simulink model "Contoh_Phoebe_2_noswitch_FIX"  (R2020b)
settings: Solver=VariableStepAuto  StartTime=0.0  StopTime=110000  FixedStep=1  RelTol=1e-3  EnableMultiTasking=on
PostLoadFcn:
  | a=find_system(gcs,'Name','Figure 1');
  | set_param(a{1},'Open','on');
  | shh = get(0,'ShowHiddenHandles');
  | set(0,'ShowHiddenHandles','On');
  | set(gcf,'Position',[500   280   546   449]);
  | set(0,'ShowHiddenHandles',shh);
InitFcn:
  | load datazr;
  | load datazl;
values from neighbouring files (symbols this model uses):
  G = 0.4*1e-5    (= 4e-06)    [initrun.m]
  k1 = 2*ze*wn*I/G    [initrun.m]
  k2 = 1    [initrun.m]
undefined symbols (not defined in the file or in its folder): gcf, outputDelta, pCalc, semimajor, set, Zl, Zr
libraries: aerolibconvert2 x2, vrlib x2, simulink x1
settings Model: Creator=Ridanto  LastModifiedBy=Asus
settings SolverCC: ZeroCrossAlgorithm=Adaptive
settings DataIOCC: LimitDataPoints=on  SaveFormat=Array  SignalLoggingSaveFormat=ModelDataLogs  ReturnWorkspaceOutputs=off
settings OptimizationCC: BufferReuse=off  ExpressionDepthLimit=2147483647  InitFltsAndDblsToZero=on  LifeSpan=inf
settings DebuggingCC: SaveWithParameterizedLinksMsg=none  UnderspecifiedInitializationDetection=Classic  MergeDetectMultiDrivingBlocksExec=none  SignalResolutionControl=TryResolveAllWithWarning  IgnoredZcDiagnostic=none  SolverPrmCheckMsg=warning  MultiTaskDSMMsg=warning  MultiTaskCondExecSysMsg=none  FcnCallInpInsideContextMsg=warning  StateNameClashWarn=warning  SFUnexpectedBacktrackingDiag=warning  SFNoUnconditionalDefaultTransitionDiag=warning  SFExecutionAtInitializationDiag=none  ArithmeticOperatorsInVariantConditions=warning
settings HardwareCC: ProdBitPerPointer=32  ProdBitPerSizeT=32  ProdBitPerPtrDiffT=32  ProdLargestAtomicFloat=None  ProdIntDivRoundTo=Undefined  ProdEndianess=Unspecified  ProdWordSize=32  ProdHWDeviceType=32-bit Generic
settings ModelReferenceCC: PropagateSignalLabelsOutOfModel=off
settings SFSimCC: SimUseLocalCustomCode=off  SimParseCustomCode=off  CustomCodeUndefinedFunction=UseInterfaceOnly
settings RTWCC: RTWUseLocalCustomCode=off
settings CodeAppCC: StateflowObjectComments=on
settings GRTTargetCC: TargetFcnLib=ansi_tfl_tmw.mat  TargetLangStandard=C89/C90 (ANSI)  CombineOutputUpdateFcns=off  GRTInterface=on
settings ConfigComp: CovMetricSettings=dw  CovSaveCumulativeToWorkspaceVar=on  CovSaveSingleToWorkspaceVar=on  CovExternalEMLEnable=off
settings SimscapeCC: SimscapeNormalizeSystem=off
settings ConfigurationSet: Description=SimMechanics 2G

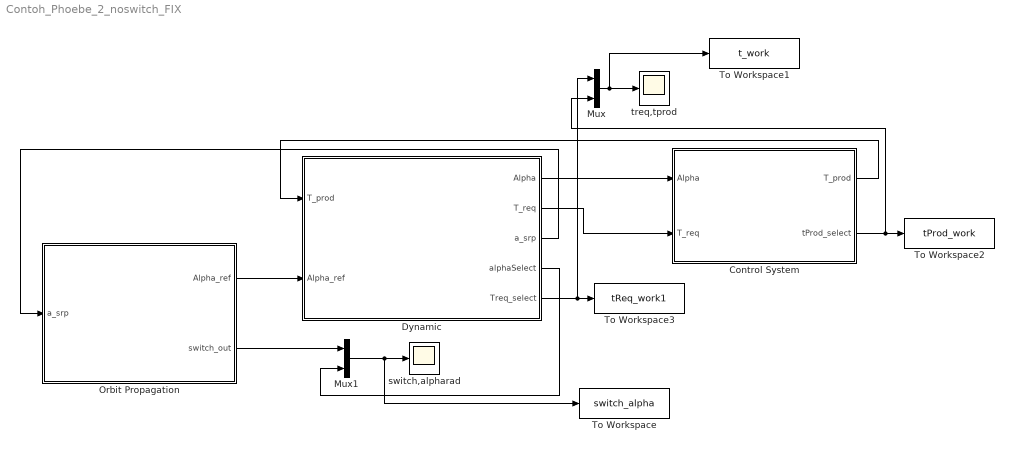
== system Contoh_Phoebe_2_noswitch_FIX ==
  Control System : Subsystem
  Dynamic : Subsystem
  Mux : Mux  Inputs=2
  Mux1 : Mux  Inputs=2
  Orbit Propagation : Subsystem
  To Workspace : ToWorkspace  VariableName=switch_alpha  SaveFormat=Timeseries  SampleTime=-1
  To Workspace1 : ToWorkspace  VariableName=t_work  SaveFormat=Timeseries  SampleTime=-1
  To Workspace2 : ToWorkspace  VariableName=tProd_work  SaveFormat=Timeseries  SampleTime=-1
  To Workspace3 : ToWorkspace  VariableName=tReq_work1  SaveFormat=Timeseries  SampleTime=-1
  switch,alpharad : Scope
  treq,tprod : Scope
  wires:
  Dynamic/2(T_req) -> Control System/2(T_req)
  Dynamic/3(a_srp) -> Orbit Propagation/1(a_srp)
  Dynamic/1(Alpha) -> Control System/1(Alpha)
  Orbit Propagation/1(Alpha_ref) -> Dynamic/2(Alpha_ref)
  Control System/1(T_prod) -> Dynamic/1(T_prod)
  Mux1/1 -> To Workspace/1, switch,alpharad/1
  Orbit Propagation/2(switch_out) -> Mux1/1
  Dynamic/4(alphaSelect) -> Mux1/2
  Mux/1 -> To Workspace1/1, treq,tprod/1
  Control System/2(tProd_select) -> Mux/2, To Workspace2/1
  Dynamic/5(Treq_select) -> Mux/1, To Workspace3/1

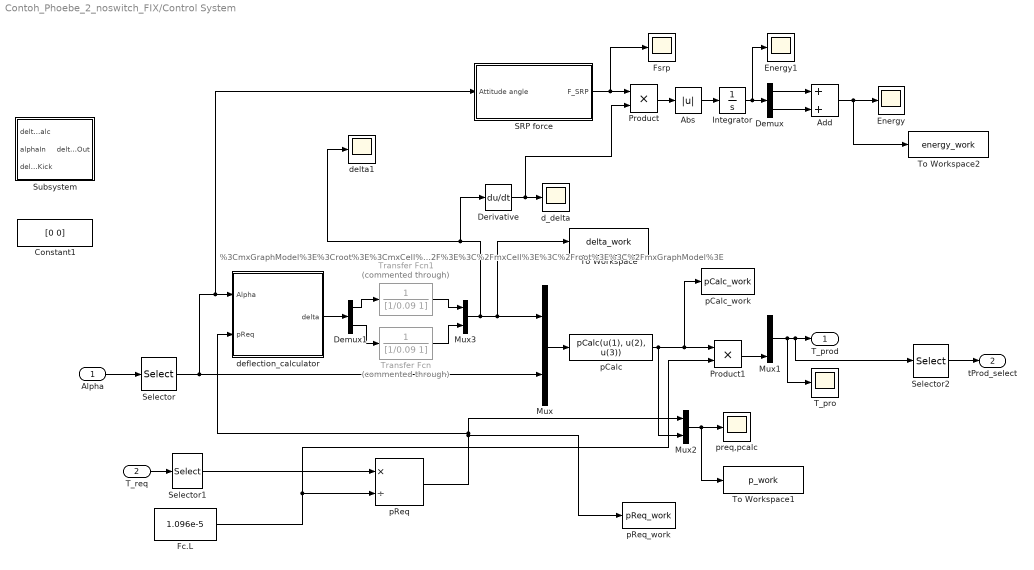
== system Contoh_Phoebe_2_noswitch_FIX/Control System ==
  note: %3CmxGraphModel%3E%3Croot%3E%3CmxCell%20id%3D%220%22%2F%3E%3CmxCell%20id%3D%221%22%20parent%3D%220%22%2F%3E%3CmxCell%20id%3D%222%22%20value%3D%22A%22%20style%3D%22ellipse%3BwhiteSpace%3Dwrap%3Bhtml%3D1%3Baspect%3Dfixed%3BfillColor%3Dnone%3B%22%20vertex%3D%221%22%20parent%3D%221%22%3E%3CmxGeometry%20x%3D%22170%22%20y%3D%221331%22%20width%3D%2260%22%20height%3D%2260%22%20as%3D%22geometry%22%2F%3E%3C%2FmxCell%3E%3C%2Froot%3E%3C%2FmxGraphModel%3E
  Alpha : Inport
  T_req : Inport  Port=2
  Abs : Abs
  Add : Sum
  Constant1 : Constant  Value=[0 0]
  Demux : Demux  Outputs=2
  Demux1 : Demux  Outputs=2
  Derivative : Derivative
  Energy : Scope
  Energy1 : Scope
  Fc.L : Constant  Value=1.096e-5
  Fsrp : Scope
  Integrator : Integrator
  Mux : Mux  Inputs=2
  Mux1 : Mux  Inputs=3
  Mux2 : Mux  Inputs=2
  Mux3 : Mux  Inputs=2
  Product : Product
  Product1 : Product
  SRP force : Subsystem
  Selector : Selector  InputPortWidth=3  IndexOptions=Index vector (dialog)  Indices=3  OutputSizes=1
  Selector1 : Selector  InputPortWidth=3  IndexOptions=Index vector (dialog)  Indices=3  OutputSizes=1
  Selector2 : Selector  InputPortWidth=3  IndexOptions=Index vector (dialog)  Indices=3  OutputSizes=1
  Subsystem : Subsystem
  T_pro : Scope
  To Workspace : ToWorkspace  VariableName=delta_work  SaveFormat=Timeseries  SampleTime=-1
  To Workspace1 : ToWorkspace  VariableName=p_work  SaveFormat=Timeseries  SampleTime=-1
  To Workspace2 : ToWorkspace  VariableName=energy_work  SaveFormat=Timeseries  SampleTime=-1
  Transfer Fcn : TransferFcn  Commented=through  Denominator=[1/0.09 1]
  Transfer Fcn1 : TransferFcn  Commented=through  Denominator=[1/0.09 1]
  d_delta : Scope
  deflection_calculator : Subsystem
  delta1 : Scope
  pCalc : MATLABFcn  MATLABFcn=pCalc(u(1), u(2), u(3))  OutputDimensions=1
  pCalc_work : ToWorkspace  VariableName=pCalc_work  SaveFormat=Timeseries  SampleTime=-1
  pReq : Product  Inputs=*/
  pReq_work : ToWorkspace  VariableName=pReq_work  SaveFormat=Timeseries  SampleTime=-1
  preq,pcalc : Scope
  T_prod : Outport
  tProd_select : Outport  Port=2
  wires:
  pReq/1 -> deflection_calculator/2(pReq), Mux2/1, pReq_work/1
  Mux1/1 -> Selector2/1, T_prod/1, T_pro/1
  Selector/1 -> Mux/2, deflection_calculator/1(Alpha), SRP force/1(Attitude angle)
  pCalc/1 -> Mux2/2, pCalc_work/1, Product1/1
  Product1/1 -> Mux1/3
  Fc.L/1 -> pReq/2, Product1/2
  Mux2/1 -> To Workspace1/1, preq,pcalc/1
  T_req/1 -> Selector1/1
  Alpha/1 -> Selector/1
  Mux/1 -> pCalc/1
  Selector1/1 -> pReq/1
  Derivative/1 -> Product/2, d_delta/1
  SRP force/1(F_SRP) -> Fsrp/1, Product/1
  Integrator/1 -> Energy1/1, Demux/1
  Demux/1 -> Add/1
  Demux/2 -> Add/2
  Add/1 -> To Workspace2/1, Energy/1
  Selector2/1 -> tProd_select/1
  Product/1 -> Abs/1
  Abs/1 -> Integrator/1
  deflection_calculator/1(delta) -> Demux1/1
  Demux1/2 -> Transfer Fcn/1
  Demux1/1 -> Transfer Fcn1/1
  Transfer Fcn1/1 -> Mux3/1
  Transfer Fcn/1 -> Mux3/2
  Mux3/1 -> delta1/1, Derivative/1, To Workspace/1, Mux/1

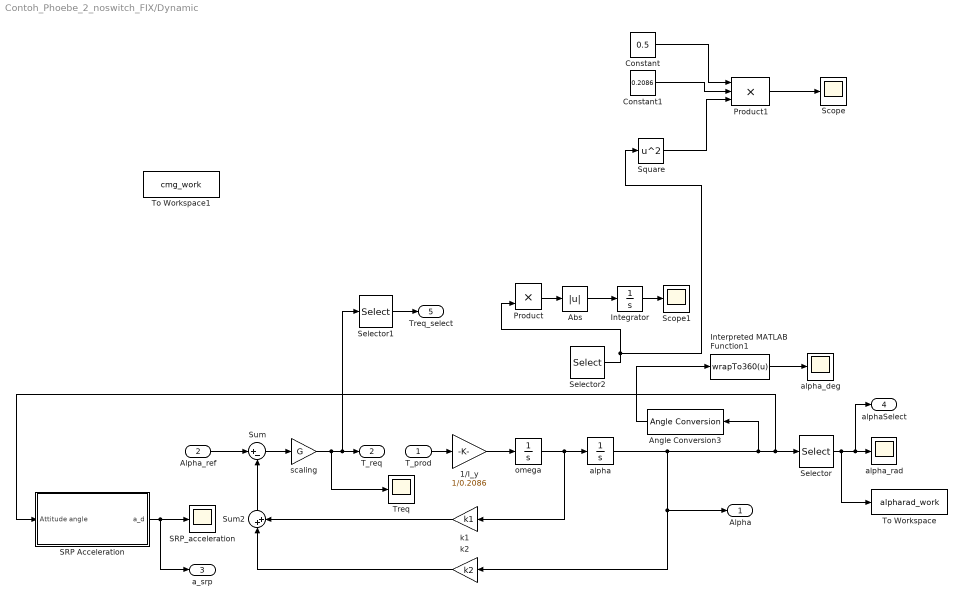
== system Contoh_Phoebe_2_noswitch_FIX/Dynamic ==
  T_prod : Inport
  Alpha_ref : Inport  Port=2
  1/I_y : Gain  Gain=1/0.2086
  Abs : Abs
  Angle Conversion3 : aerolibconvert2/Angle Conversion  IU=rad  OU=deg
  Constant : Constant  Value=0.5
  Constant1 : Constant  Value=0.2086
  Integrator : Integrator
  Interpreted MATLAB Function1 : MATLABFcn  MATLABFcn=wrapTo360(u)  OutputDimensions=3
  Product : Product
  Product1 : Product  Inputs=3
  SRP Acceleration : Subsystem
  SRP_acceleration : Scope
  Scope : Scope
  Scope1 : Scope
  Selector : Selector  InputPortWidth=3  IndexOptions=Index vector (dialog)  Indices=3  OutputSizes=1
  Selector1 : Selector  InputPortWidth=3  IndexOptions=Index vector (dialog)  Indices=3  OutputSizes=1
  Selector2 : Selector  InputPortWidth=3  IndexOptions=Index vector (dialog)  Indices=3  OutputSizes=1
  Square : Math  Operator=square  SaturateOnIntegerOverflow=on
  Sum : Sum  Inputs=|+-
  Sum2 : Sum  Inputs=|++
  To Workspace : ToWorkspace  VariableName=alpharad_work  SaveFormat=Timeseries  SampleTime=-1
  To Workspace1 : ToWorkspace  VariableName=cmg_work  SaveFormat=Timeseries  SampleTime=-1
  Treq : Scope
  alpha : Integrator  WrapState=on
  alpha_deg : Scope
  alpha_rad : Scope
  k1 : Gain  Gain=k1
  k2 : Gain  Gain=k2
  omega : Integrator
  scaling : Gain  Gain=G
  Alpha : Outport
  T_req : Outport  Port=2
  a_srp : Outport  Port=3
  alphaSelect : Outport  Port=4
  Treq_select : Outport  Port=5
  wires:
  Interpreted MATLAB Function1/1 -> alpha_deg/1
  k2/1 -> Sum2/1
  Sum2/1 -> Sum/2
  SRP Acceleration/1(a_d) -> a_srp/1, SRP_acceleration/1
  1/I_y/1 -> omega/1
  k1/1 -> Sum2/2
  Angle Conversion3/1 -> Interpreted MATLAB Function1/1
  Alpha_ref/1 -> Sum/1
  Sum/1 -> scaling/1
  alpha/1 -> Selector/1, SRP Acceleration/1(Attitude angle), Angle Conversion3/1, Alpha/1, k2/1
  Selector/1 -> To Workspace/1, alphaSelect/1, alpha_rad/1
  Selector1/1 -> Treq_select/1
  scaling/1 -> T_req/1, Selector1/1, Treq/1
  omega/1 -> alpha/1, k1/1
  Constant1/1 -> Product1/2
  Constant/1 -> Product1/1
  Product1/1 -> Scope/1
  Square/1 -> Product1/3
  Abs/1 -> Integrator/1
  Product/1 -> Abs/1
  Integrator/1 -> Scope1/1
  Selector2/1 -> Square/1, Product/2
  T_prod/1 -> 1/I_y/1

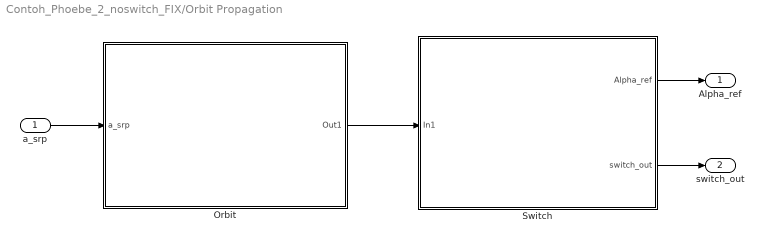
== system Contoh_Phoebe_2_noswitch_FIX/Orbit Propagation ==
  a_srp : Inport
  "Orbit " : Subsystem
  Switch : Subsystem
  Alpha_ref : Outport
  switch_out : Outport  Port=2
  wires:
  "Orbit "/1(Out1) -> Switch/1(In1)
  a_srp/1 -> "Orbit "/1(a_srp)
  Switch/1(Alpha_ref) -> Alpha_ref/1
  Switch/2(switch_out) -> switch_out/1

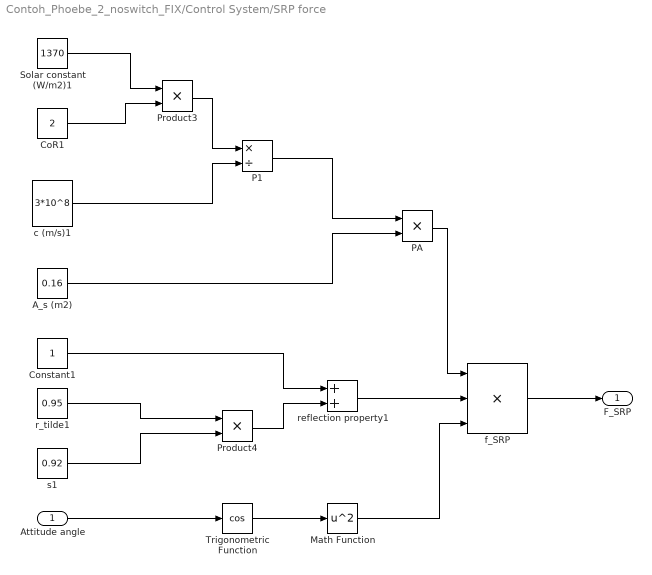
== system Contoh_Phoebe_2_noswitch_FIX/Control System/SRP force ==
  Attitude angle : Inport
  A_s (m2) : Constant  Value=0.16
  CoR1 : Constant  Value=2
  Constant1 : Constant
  Math Function : Math  Operator=square  SaturateOnIntegerOverflow=on
  P1 : Product  Inputs=*/
  PA : Product
  Product3 : Product
  Product4 : Product
  Solar constant (W/m2)1 : Constant  Value=1370
  Trigonometric Function : Trigonometry  Operator=cos
  c (m/s)1 : Constant  Value=3*10^8
  f_SRP : Product  Inputs=3
  r_tilde1 : Constant  Value=0.95
  reflection property1 : Sum
  s1 : Constant  Value=0.92
  F_SRP : Outport
  wires:
  A_s (m2)/1 -> PA/2
  Solar constant (W/m2)1/1 -> Product3/1
  r_tilde1/1 -> Product4/1
  CoR1/1 -> Product3/2
  s1/1 -> Product4/2
  Math Function/1 -> f_SRP/3
  c (m/s)1/1 -> P1/2
  PA/1 -> f_SRP/1
  Constant1/1 -> reflection property1/1
  Product3/1 -> P1/1
  P1/1 -> PA/1
  reflection property1/1 -> f_SRP/2
  Trigonometric Function/1 -> Math Function/1
  Product4/1 -> reflection property1/2
  f_SRP/1 -> F_SRP/1
  Attitude angle/1 -> Trigonometric Function/1

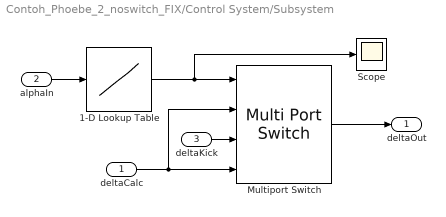
== system Contoh_Phoebe_2_noswitch_FIX/Control System/Subsystem ==
  deltaCalc : Inport
  alphaIn : Inport  Port=2
  deltaKick : Inport  Port=3
  1-D Lookup Table : Lookup_n-D  NumberOfTableDimensions=1  BreakpointsForDimension1=deg2rad([-1 1 89 91])  Table=[1 2 1 1]  InterpMethod=Flat  InternalRulePriority=Speed  RndMeth=Simplest  InputSameDT=on
  Multiport Switch : MultiPortSwitch  Inputs=2  DataPortForDefault=Additional data port
  Scope : Scope
  deltaOut : Outport
  wires:
  Multiport Switch/1 -> deltaOut/1
  alphaIn/1 -> 1-D Lookup Table/1
  deltaCalc/1 -> Multiport Switch/2, Multiport Switch/4
  deltaKick/1 -> Multiport Switch/3
  1-D Lookup Table/1 -> Scope/1, Multiport Switch/1

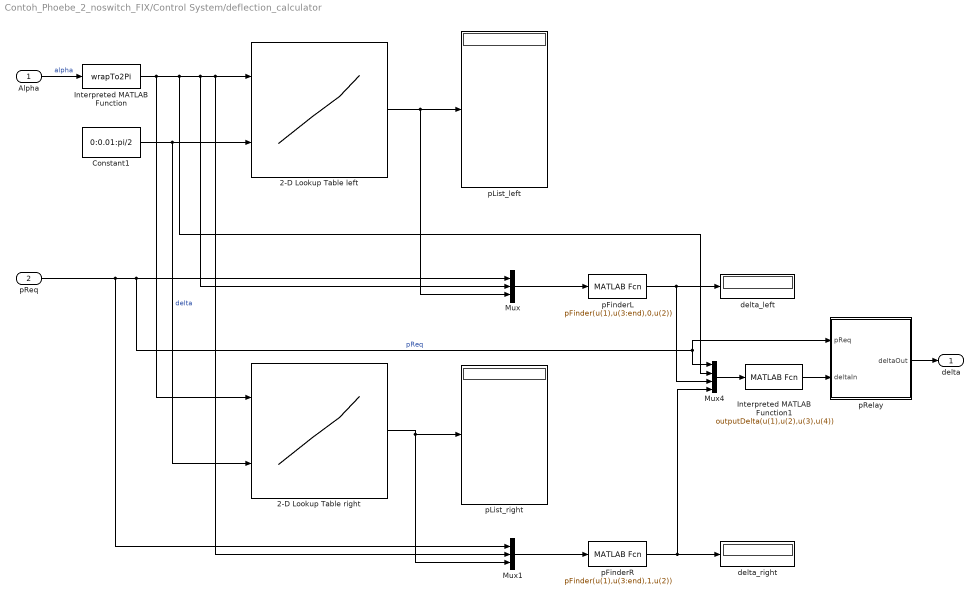
== system Contoh_Phoebe_2_noswitch_FIX/Control System/deflection_calculator ==
  Alpha : Inport
  pReq : Inport  Port=2
  2-D Lookup Table left : Lookup_n-D  BreakpointsForDimension1=0:0.01:2*pi  BreakpointsForDimension2=0:0.01:pi/2  IndexSearchMethod=Linear search  Table=Zl  InternalRulePriority=Speed  RndMeth=Simplest  InputSameDT=on
      settings: InputPortMap=u0,u1
  2-D Lookup Table right : Lookup_n-D  BreakpointsForDimension1=0:0.01:2*pi  BreakpointsForDimension2=0:0.01:pi/2  IndexSearchMethod=Linear search  Table=Zr  InternalRulePriority=Speed  RndMeth=Simplest  InputSameDT=on
      settings: InputPortMap=u0,u1
  Constant1 : Constant  Value=0:0.01:pi/2
  Interpreted MATLAB Function : MATLABFcn  MATLABFcn=wrapTo2Pi
  Interpreted MATLAB Function1 : MATLABFcn  MATLABFcn=outputDelta(u(1),u(2),u(3),u(4))
  Mux : Mux  Inputs=3
  Mux1 : Mux  Inputs=3
  Mux4 : Mux
  delta_left : Display
  delta_right : Display
  pFinderL : MATLABFcn  MATLABFcn=pFinder(u(1),u(3:end),0,u(2))
  pFinderR : MATLABFcn  MATLABFcn=pFinder(u(1),u(3:end),1,u(2))
  pList_left : Display
  pList_right : Display
  pRelay : Subsystem
  delta : Outport
  wires:
  pReq/1 -> Mux1/1, Mux4/1, pRelay/1(pReq), Mux/1  "pReq"
  Alpha/1 -> Interpreted MATLAB Function/1  "alpha"
  Mux/1 -> pFinderL/1
  2-D Lookup Table left/1 -> Mux/3, pList_left/1
  pFinderR/1 -> delta_right/1, Mux4/4
  pFinderL/1 -> delta_left/1, Mux4/3
  2-D Lookup Table right/1 -> Mux1/3, pList_right/1
  Mux1/1 -> pFinderR/1
  Constant1/1 -> 2-D Lookup Table left/2, 2-D Lookup Table right/2  "delta"
  Interpreted MATLAB Function/1 -> 2-D Lookup Table right/1, Mux4/2, Mux/2, Mux1/2, 2-D Lookup Table left/1
  Mux4/1 -> Interpreted MATLAB Function1/1
  Interpreted MATLAB Function1/1 -> pRelay/2(deltaIn)
  pRelay/1(deltaOut) -> delta/1

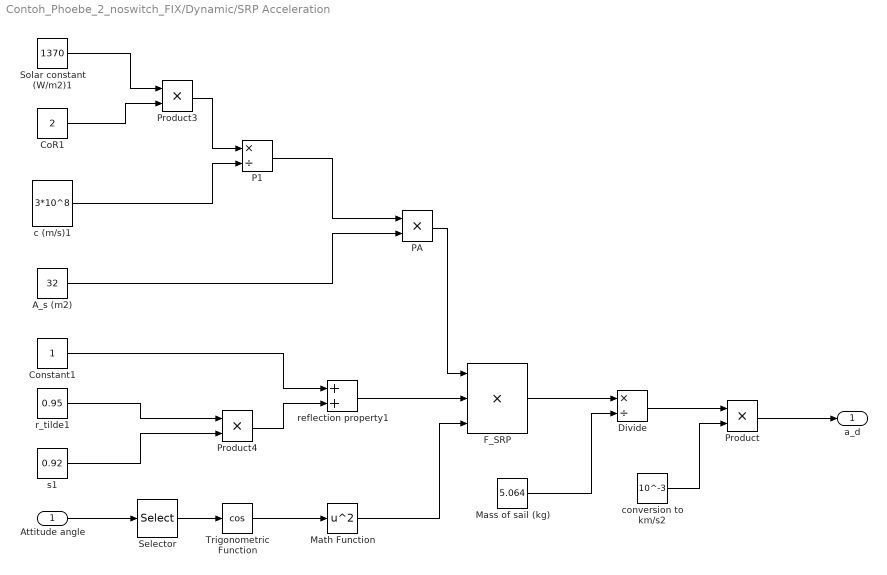
== system Contoh_Phoebe_2_noswitch_FIX/Dynamic/SRP Acceleration ==
  Attitude angle : Inport
  A_s (m2) : Constant  Value=32
  CoR1 : Constant  Value=2
  Constant1 : Constant
  Divide : Product  Inputs=*/
  F_SRP : Product  Inputs=3
  Mass of sail (kg) : Constant  Value=5.064
  Math Function : Math  Operator=square  SaturateOnIntegerOverflow=on
  P1 : Product  Inputs=*/
  PA : Product
  Product : Product
  Product3 : Product
  Product4 : Product
  Selector : Selector  InputPortWidth=3  IndexOptions=Index vector (dialog)  Indices=3  OutputSizes=1
  Solar constant (W/m2)1 : Constant  Value=1370
  Trigonometric Function : Trigonometry  Operator=cos
  c (m/s)1 : Constant  Value=3*10^8
  conversion to km/s2 : Constant  Value=10^-3
  r_tilde1 : Constant  Value=0.95
  reflection property1 : Sum
  s1 : Constant  Value=0.92
  a_d : Outport
  wires:
  A_s (m2)/1 -> PA/2
  Solar constant (W/m2)1/1 -> Product3/1
  r_tilde1/1 -> Product4/1
  CoR1/1 -> Product3/2
  s1/1 -> Product4/2
  Math Function/1 -> F_SRP/3
  c (m/s)1/1 -> P1/2
  PA/1 -> F_SRP/1
  Constant1/1 -> reflection property1/1
  Product3/1 -> P1/1
  P1/1 -> PA/1
  reflection property1/1 -> F_SRP/2
  Attitude angle/1 -> Selector/1
  Trigonometric Function/1 -> Math Function/1
  Product4/1 -> reflection property1/2
  F_SRP/1 -> Divide/1
  Mass of sail (kg)/1 -> Divide/2
  conversion to km/s2/1 -> Product/2
  Divide/1 -> Product/1
  Product/1 -> a_d/1
  Selector/1 -> Trigonometric Function/1

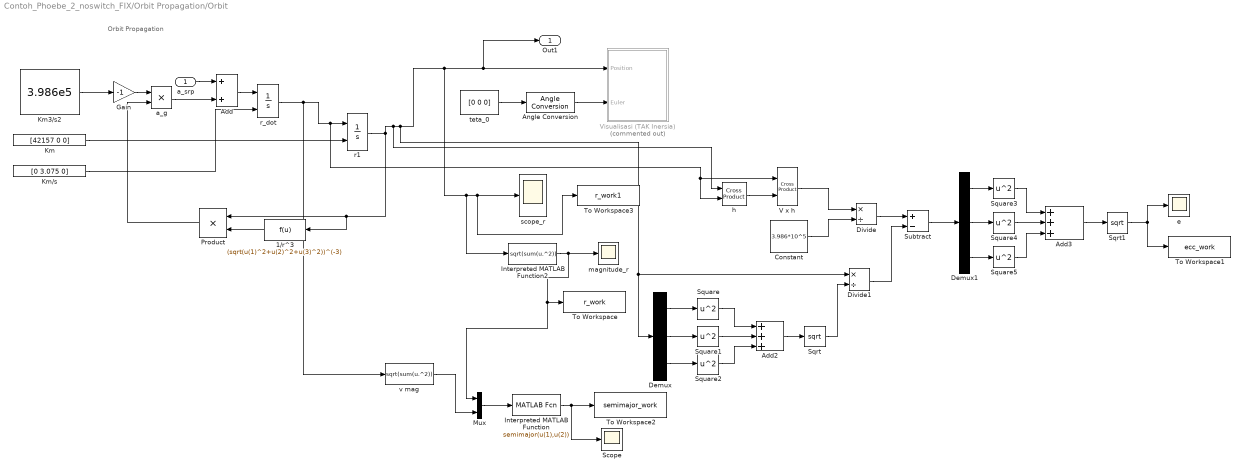
== system Contoh_Phoebe_2_noswitch_FIX/Orbit Propagation/Orbit  ==
  note: Orbit Propagation
  a_srp : Inport
  1/r^3 : Fcn  Expr=(sqrt(u(1)^2+u(2)^2+u(3)^2))^(-3)
  Add : Sum
  Add2 : Sum  Inputs=3
  Add3 : Sum  Inputs=3
  Angle Conversion : aerolibconvert2/Angle Conversion  IU=deg  OU=rad
  Constant : Constant  Value=3.986*10^5
  Demux : Demux  Outputs=3
  Demux1 : Demux  Outputs=3
  Divide : Product  Inputs=*/
  Divide1 : Product  Inputs=*/
  Gain : Gain  Gain=-1
  Interpreted MATLAB Function : MATLABFcn  MATLABFcn=semimajor(u(1),u(2))
  Interpreted MATLAB Function2 : MATLABFcn  MATLABFcn=sqrt(sum(u.^2))
  Km : Constant  Value=[42157 0 0]
  Km/s : Constant  Value=[0 3.075 0]
  Km3/s2 : Constant  Value=3.986e5
  Mux : Mux  Inputs=2
  Product : Product  RndMeth=Zero
  Scope : Scope
  Sqrt : Sqrt  SaturateOnIntegerOverflow=on
  Sqrt1 : Sqrt  SaturateOnIntegerOverflow=on
  Square{,1..5} (6 alike) : Math  Operator=square  SaturateOnIntegerOverflow=on
  Subtract : Sum  Inputs=+-
  To Workspace : ToWorkspace  VariableName=r_work  SaveFormat=Timeseries  SampleTime=-1
  To Workspace1 : ToWorkspace  VariableName=ecc_work  SaveFormat=Timeseries  SampleTime=-1
  To Workspace2 : ToWorkspace  VariableName=semimajor_work  SaveFormat=Timeseries  SampleTime=-1
  To Workspace3 : ToWorkspace  VariableName=r_work1  SaveFormat=Timeseries  SampleTime=-1
  V x h : vrlib/Utilities/Cross Product
  Visualisasi (TAK Inersia) : Subsystem  Commented=on  StartFcn=set(gcf,'Position',[18 57 324 239]);  mask(6DoF_Animation){u1=[-100000 100000 -100000 100000 -100000 100000], u2=2, u3=3000, u4=[0 0 0], u5=Fixed Position, u6=[60000 70000 60000], u7=30, u8=on}
      mask prompts: u1 "Axes limits [xmin xmax ymin ymax zmin zmax]:"; u2 "Time interval between updates:"; u3 "Size of craft displayed:"; u4 "Static object position [xp yp zp]:"; u5 "Enter view:"; u6 "Position of camera [xc yc zc]:"; u7 "View angle:"; u8 "Enable animation"
      mask init:
      | Config.axes = u1;
      | Config.update = u2;
      | Config.craft = u3;
      | Config.target = u4;
      | Config.camera_view = u5;
      | Config.camera_pos = u6;
      | Config.view = u7;
      | Config.Animenable = u8;
      | Config.Model = bdroot(gcb);
      mask TypeOptions u5: Fixed Position | Cockpit | Fly alongside
      mask Display:
      | port_label('input',1,'x_e','texmode','on');
      | port_label('input',2,'\phi \theta \psi','texmode','on');
      | [xp yp] = aeroimage('anim',gcbh);
      | patch(xp,yp)
  a_g : Product  RndMeth=Zero
  e : Scope
  h : vrlib/Utilities/Cross Product
  magnitude_r : Scope
  r1 : Integrator  InitialConditionSource=external
  r_dot : Integrator  InitialConditionSource=external  InitialCondition=8
  scope_r : Scope
  teta_0 : Constant  Value=[0 0 0]
  v mag : MATLABFcn  MATLABFcn=sqrt(sum(u.^2))
  Out1 : Outport
  wires:
  Gain/1 -> a_g/1
  r_dot/1 -> V x h/1, h/2, r1/1, v mag/1
  Add/1 -> r_dot/1
  Interpreted MATLAB Function2/1 -> Mux/1, To Workspace/1, magnitude_r/1
  Add2/1 -> Sqrt/1
  V x h/1 -> Divide/1
  Square3/1 -> Add3/1
  teta_0/1 -> Angle Conversion/1
  Square5/1 -> Add3/3
  Square1/1 -> Add2/2
  Add3/1 -> Sqrt1/1
  Demux/2 -> Square1/1
  Subtract/1 -> Demux1/1
  Sqrt/1 -> Divide1/2
  Km/s/1 -> r_dot/2
  Divide/1 -> Subtract/1
  Product/1 -> a_g/2
  Demux1/3 -> Square5/1
  Sqrt1/1 -> e/1, To Workspace1/1
  Square4/1 -> Add3/2
  Angle Conversion/1 -> Visualisasi (TAK Inersia)/2(Euler)
  1/r^3/1 -> Product/2
  r1/1 -> h/1, Divide1/1, Demux/1, Out1/1, Visualisasi (TAK Inersia)/1(Position), Interpreted MATLAB Function2/1, To Workspace3/1, scope_r/1, 1/r^3/1, Product/1
  Square/1 -> Add2/1
  Constant/1 -> Divide/2
  Demux1/2 -> Square4/1
  Km/1 -> r1/2
  Km3/s2/1 -> Gain/1
  Demux/1 -> Square/1
  Demux/3 -> Square2/1
  Square2/1 -> Add2/3
  a_g/1 -> Add/2
  h/1 -> V x h/2
  Demux1/1 -> Square3/1
  Divide1/1 -> Subtract/2
  a_srp/1 -> Add/1
  v mag/1 -> Mux/2
  Mux/1 -> Interpreted MATLAB Function/1
  Interpreted MATLAB Function/1 -> Scope/1, To Workspace2/1

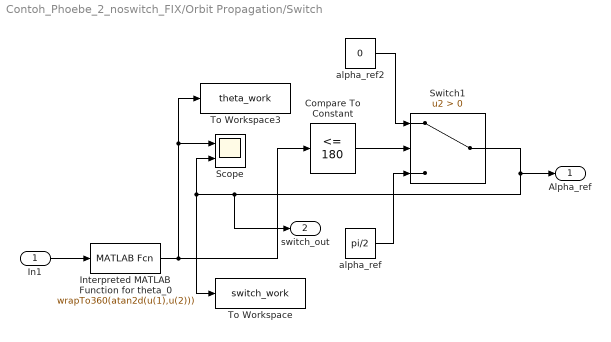
== system Contoh_Phoebe_2_noswitch_FIX/Orbit Propagation/Switch ==
  In1 : Inport
  Compare To Constant : simulink/Logic and Bit Operations/Compare To Constant  relop=<=  const=180  OutDataTypeStr=boolean
  Interpreted MATLAB Function for theta_0 : MATLABFcn  MATLABFcn=wrapTo360(atan2d(u(1),u(2)))  OutputDimensions=1
  Scope : Scope  NumInputPorts=2
  Switch1 : Switch  Criteria=u2 > Threshold
  To Workspace : ToWorkspace  VariableName=switch_work  SaveFormat=Timeseries  SampleTime=-1
  To Workspace3 : ToWorkspace  VariableName=theta_work  SaveFormat=Timeseries  SampleTime=-1
  alpha_ref : Constant  Value=pi/2
  alpha_ref2 : Constant  Value=0
  Alpha_ref : Outport
  switch_out : Outport  Port=2
  wires:
  Switch1/1 -> switch_out/1, Scope/2, To Workspace/1, Alpha_ref/1
  alpha_ref2/1 -> Switch1/1
  Compare To Constant/1 -> Switch1/2
  Interpreted MATLAB Function for theta_0/1 -> Compare To Constant/1, To Workspace3/1, Scope/1
  alpha_ref/1 -> Switch1/3
  In1/1 -> Interpreted MATLAB Function for theta_0/1

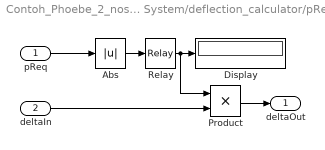
== system Contoh_Phoebe_2_noswitch_FIX/Control System/deflection_calculator/pRelay ==
  pReq : Inport
  deltaIn : Inport  Port=2
  Abs : Abs  ZeroCross=off
  Display : Display
  Product : Product
  Relay : Relay  OnSwitchValue=0.0007  OffSwitchValue=0.0007  ZeroCross=off
  deltaOut : Outport
  wires:
  pReq/1 -> Abs/1
  Abs/1 -> Relay/1
  Relay/1 -> Product/1, Display/1
  Product/1 -> deltaOut/1
  deltaIn/1 -> Product/2

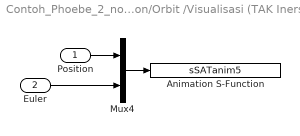
== system Contoh_Phoebe_2_noswitch_FIX/Orbit Propagation/Orbit /Visualisasi (TAK Inersia) ==
  Position : Inport
  Euler : Inport  Port=2
  Animation S-Function : S-Function  FunctionName=sSATanim5  Parameters=Config  SFunctionDeploymentMode=off  EnableBusSupport=off
  Mux4 : Mux  Inputs=2
  wires:
  Position/1 -> Mux4/1
  Mux4/1 -> Animation S-Function/1
  Euler/1 -> Mux4/2
